simulink model "B2B_2x15kW_LCO_paralelo_y_serie"  (R2026b)
settings: Solver=ode5  StopTime=inf  EnableMultiTasking=on
StopFcn:
  | Modelo_Disable_B2B
undefined symbols (not defined in the file): ALPHA_DC, COS_RO, dataStateMachine, DiscIntNeverNeededParam, dq2abc, EN_G, getNormalizedOffset, I_MAX_G, INV_SIN_RO, KAW_CCG, KAW_DC, KI_CCG, KI_DC, KI_PLLG, KP_CCG, KP_DC, KP_PLLG, L12, LIMIT_SAG_DETECT, magnitude, MIN_VDC_READY, Ncount, NDELAY_SAG_DETECT, PORC_DC_STEADS, SAMPLES_SAG_DETECT, simDCcontCurrent1, simDCcontCurrent2, SN_G, Transformations_blocks, ts, Ts_al, TS_C, TS_PLL, UDC_min_al, UDC_Ref_al, VDC_REF, WN_G
libraries: simulink x15, TriPhaseDriveControl x13, powerlib_extras x2, model_hardware_PM15F80C_rev x2, TriphaseXenomaiTarget x1
(part 4 of 4)

== matlab function B2B_2x15kW_LCO_paralelo_y_serie/VSC2 Controller/State Machine/State Machine ==
  settings: fimath=|
      | fimath(...
      | 'RoundMode', 'floor',...
      | 'OverflowMode', 'wrap',...
      | 'ProductMode', 'KeepLSB', 'ProductWordLength', 32,...
      | 'SumMode', 'KeepLSB', 'SumWordLength', 32,...
      | 'CastBeforeSum', false)
  data: data input; outputs output; nowState output; nowCounters output; inputs input size=6; prevState input; prevCounters input
function [outputs, nowState, nowCounters] = fcn(data, inputs, prevState, prevCounters)

%%%%%%%%%%%%%%%%%%%%%%%%%%%%%%%%%%%%%%%%%%%%%%%%%%%%%%%%%%%%%%%%%%%%%%%%%%%
%List of states
%%%%%%%%%%%%%%%%%%%%%%%%%%%%%%%%%%%%%%%%%%%%%%%%%%%%%%%%%%%%%%%%%%%%%%%%%%%

%1: POWER_ON              : Power on, everything deactivated
%2: PRECHARGE             : Precharge of the DC-link capacitors
%3: STANDBY               : Waiting to start
%4: START                 : Start sequence 
%5: OPERATING             : Normal operation 

%Initial value
state = prevState;

%%%%%%%%%%%%%%%%%%%%%%%%%%%%%%%%%%%%%%%%%%%%%%%%%%%%%%%%%%%%%%%%%%%%%%%%%%%
%List of data
%%%%%%%%%%%%%%%%%%%%%%%%%%%%%%%%%%%%%%%%%%%%%%%%%%%%%%%%%%%%%%%%%%%%%%%%%%%

%1: Nprecharge
%2: Nconnect
%3: NinitCCG

%Set the data to variables
Nprecharge   = data(1);
Nconnect     = data(2);
NinitCCG     = data(3);

%%%%%%%%%%%%%%%%%%%%%%%%%%%%%%%%%%%%%%%%%%%%%%%%%%%%%%%%%%%%%%%%%%%%%%%%%%%
%List of Inputs
%%%%%%%%%%%%%%%%%%%%%%%%%%%%%%%%%%%%%%%%%%%%%%%%%%%%%%%%%%%%%%%%%%%%%%%%%%%

%1:  PRECHARGE         : 0 NO precharge required
%                      : 1 
%2:  CONNECT           : 0 NO connection required
%                      : 1
%3:  SEL_QVCONTROL     : 0 V controller
%                      : 1 Q controller
%4:  VDC_READY         : 0 VDV >= than stablished value
%                      : 1 
%5:  VDC_STEADS        : 0 Not reached DC steady-state
%                      : 1 
%6:  FLAG_SAG          : 0 No voltage sag detected
%                      : 1 

%Set the variables to its names
PRECHARGE     = inputs(1);
CONNECT       = inputs(2);
SEL_QVCONTROL = inputs(3);
VDC_READY     = inputs(4);
VDC_STEADS    = inputs(5);
FLAG_SAG      = inputs(6);

%%%%%%%%%%%%%%%%%%%%%%%%%%%%%%%%%%%%%%%%%%%%%%%%%%%%%%%%%%%%%%%%%%%%%%%%%%%
%List of outputs
%%%%%%%%%%%%%%%%%%%%%%%%%%%%%%%%%%%%%%%%%%%%%%%%%%%%%%%%%%%%%%%%%%%%%%%%%%%

%PWMOnGrid                     : 0 Do NOT PWM of grid converter
%                              : 1 
%CONNECT_GRID_CONTACT          : 0 NO connection to grid
%                              : 1
%CONNECT_PRELOAD_CONTACT       : 0 NO connection of precharge
%                              : 1 
%selReactiveVoltageController  : 0 Selection of V control
%                              : 1 Selection of Q control
%initPLLGrid                   : 0 Do NOT activate the PLL
%                              : 1 
%initReactiveVoltageController : 0 NO activate the external AC control (Q/VAC)
%                              : 1
%initCurrentControllerG        : 0 Do NOT initilialise the current controller
%                              : 1 
%initDCControllerGrid          : 0 Do NOT initialise the DC controller
%                              : 1                        

%Initilisation
PWMOnGrid               = 0;
CONNECT_GRID_CONTACT    = 0;
CONNECT_PRELOAD_CONTACT = 0;
selReactiveVoltageController  = SEL_QVCONTROL;
initPLLGrid             = 0;
initReactiveVoltageController = 0;
initCurrentControllerG  = 0;
initDCControllerGrid    = 0;

%%%%%%%%%%%%%%%%%%%%%%%%%%%%%%%%%%%%%%%%%%%%%%%%%%%%%%%%%%%%%%%%%%%%%%%%%%%
%List of counters
%%%%%%%%%%%%%%%%%%%%%%%%%%%%%%%%%%%%%%%%%%%%%%%%%%%%%%%%%%%%%%%%%%%%%%%%%%%

%Initilisation
CONT_PRECHARGE   = 0;
CONT_CONNECT     = 0;
CONT_INIT_CC     = 0;

%Adjustment of vector counters
CONT_PRECHARGE_ANT   = prevCounters(1);
CONT_CONNECT_ANT     = prevCounters(2);
CONT_INIT_CC_ANT     = prevCounters(3);

%%%%%%%%%%%%%%%%%%%%%%%%%%%%%%%%%%%%%%%%%%%%%%%%%%%%%%%%%%%%%%%%%%%%%%%%%%%
%STATE MACHINE: MAIN SWITCH
%%%%%%%%%%%%%%%%%%%%%%%%%%%%%%%%%%%%%%%%%%%%%%%%%%%%%%%%%%%%%%%%%%%%%%%%%%%

switch prevState

%%%%%%%%%%%%%%%%%%%%%%%%%%%%%%%%%%%%%%%%%%%%%%%%%%%%%%%%%%%%%%%%%%%%%%%%%%%
%STATE 1: POWER_ON
%%%%%%%%%%%%%%%%%%%%%%%%%%%%%%%%%%%%%%%%%%%%%%%%%%%%%%%%%%%%%%%%%%%%%%%%%%%

case 1

%Outputs for the state
PWMOnGrid               = 0;
CONNECT_GRID_CONTACT    = 0;
CONNECT_PRELOAD_CONTACT = 0;
selReactiveVoltageController  = SEL_QVCONTROL;
initPLLGrid             = 0;
initReactiveVoltageController = 0;
initDCControllerGrid    = 0;

%Counter initialisation
CONT_PRECHARGE   = 0;
CONT_CONNECT     = 0;
CONT_INIT_CC     = 0;

%Conditions to change state
if (PRECHARGE == 1) %Precharge
    state = 2;                            %Change to state 2 
end

%%%%%%%%%%%%%%%%%%%%%%%%%%%%%%%%%%%%%%%%%%%%%%%%%%%%%%%%%%%%%%%%%%%%%%%%%%%
%STATE 2: PRECHARGE
%%%%%%%%%%%%%%%%%%%%%%%%%%%%%%%%%%%%%%%%%%%%%%%%%%%%%%%%%%%%%%%%%%%%%%%%%%%

case 2

%Outputs for the state
PWMOnGrid               = 0;
CONNECT_GRID_CONTACT    = 0;
CONNECT_PRELOAD_CONTACT = 1;
selReactiveVoltageController = SEL_QVCONTROL;
initPLLGrid             = 1;
initReactiveVoltageController = 0;
initCurrentControllerG  = 0;
initDCControllerGrid    = 0;

%Counter initialisation
CONT_PRECHARGE   = 1;
CONT_CONNECT     = 0;
CONT_INIT_CC     = 0;

%Conditions to change state
if (PRECHARGE == 0) %If precharge is zero, go init
    state = 1;
end

if ((CONT_PRECHARGE_ANT >= Nprecharge) && (VDC_READY == 1)) % If time for precharge is reached
    state = 3;              %Go to standby
    CONT_PRECHARGE_ANT = 0; %Unload the counter
end

%%%%%%%%%%%%%%%%%%%%%%%%%%%%%%%%%%%%%%%%%%%%%%%%%%%%%%%%%%%%%%%%%%%%%%%%%%%
%STATE 3: STANDBY
%%%%%%%%%%%%%%%%%%%%%%%%%%%%%%%%%%%%%%%%%%%%%%%%%%%%%%%%%%%%%%%%%%%%%%%%%%%

case 3

%Outputs for the state
PWMOnGrid               = 0;
CONNECT_GRID_CONTACT    = 1;
CONNECT_PRELOAD_CONTACT = 0;
selReactiveVoltageController = SEL_QVCONTROL;
initPLLGrid             = 1;
initReactiveVoltageController = 0;
initCurrentControllerG  = 0;
initDCControllerGrid    = 0;

%Counter initialisation
CONT_PRECHARGE   = 0;
CONT_CONNECT     = 1;
CONT_INIT_CC     = 0;

%Conditions to change state
if ((CONT_CONNECT_ANT >= Nconnect) && (CONNECT == 1) && (VDC_STEADS == 1)) %If time to connect is reached
	state = 4; 
    CONT_CONNECT_ANT = 0; %Unload the counter
end

%%%%%%%%%%%%%%%%%%%%%%%%%%%%%%%%%%%%%%%%%%%%%%%%%%%%%%%%%%%%%%%%%%%%%%%%%%%
%STATE 4: START
%%%%%%%%%%%%%%%%%%%%%%%%%%%%%%%%%%%%%%%%%%%%%%%%%%%%%%%%%%%%%%%%%%%%%%%%%%%

case 4

%Outputs for the state
PWMOnGrid               = 1;
CONNECT_GRID_CONTACT    = 1;
CONNECT_PRELOAD_CONTACT = 0;
selReactiveVoltageController = SEL_QVCONTROL;
initPLLGrid             = 1;
initReactiveVoltageController = 0;
initCurrentControllerG  = 1;
initDCControllerGrid    = 1;

%Counter initialisation
CONT_PRECHARGE   = 0;
CONT_CONNECT     = 0;
CONT_INIT_CC     = 1;

%Conditions to change state
if (CONT_INIT_CC_ANT >= NinitCCG)  %If time to start is reached
    state = 5;                     %Go to regular operation
    CONT_INIT_CC_ANT = 0;          %Unload the counter
end

if (CONNECT == 0)  %If connect equals zero
    state = 1;     %Dischonnect
end

%%%%%%%%%%%%%%%%%%%%%%%%%%%%%%%%%%%%%%%%%%%%%%%%%%%%%%%%%%%%%%%%%%%%%%%%%%%
%STATE 5: OPERATING
%%%%%%%%%%%%%%%%%%%%%%%%%%%%%%%%%%%%%%%%%%%%%%%%%%%%%%%%%%%%%%%%%%%%%%%%%%%

case 5

%Outputs for the state
PWMOnGrid               = 1;
CONNECT_GRID_CONTACT    = 1;
CONNECT_PRELOAD_CONTACT = 0;
selReactiveVoltageController = SEL_QVCONTROL;
initPLLGrid             = 1;
initReactiveVoltageController = 1;
initCurrentControllerG  = 1;
initDCControllerGrid    = 1;

%Counter initialisation
CONT_PRECHARGE   = 0;
CONT_CONNECT     = 0;
CONT_INIT_CC     = 0;

%Conditions to change state
if (CONNECT == 0)  %If connect equals zero
    state = 1;     %Dischonnect
end

%%%%%%%%%%%%%%%%%%%%%%%%%%%%%%%%%%%%%%%%%%%%%%%%%%%%%%%%%%%%%%%%%%%%%%%%%%%
%STATE MACHINE: END STATE MACHINE
%%%%%%%%%%%%%%%%%%%%%%%%%%%%%%%%%%%%%%%%%%%%%%%%%%%%%%%%%%%%%%%%%%%%%%%%%%%

end 

%%%%%%%%%%%%%%%%%%%%%%%%%%%%%%%%%%%%%%%%%%%%%%%%%%%%%%%%%%%%%%%%%%%%%%%%%%%
%INCREASE AND RESET COUNTERS
%%%%%%%%%%%%%%%%%%%%%%%%%%%%%%%%%%%%%%%%%%%%%%%%%%%%%%%%%%%%%%%%%%%%%%%%%%%

%PRECHARGE counter
if (CONT_PRECHARGE == 1)
    CONT_PRECHARGE = CONT_PRECHARGE_ANT + CONT_PRECHARGE;
else
    CONT_PRECHARGE = 0;
end

%CONNECT counter
if (CONT_CONNECT == 1)
    CONT_CONNECT = CONT_CONNECT_ANT + CONT_CONNECT;
else
    CONT_CONNECT = 0;
end

%INIT_CC counter
if (CONT_INIT_CC == 1)
    CONT_INIT_CC = CONT_INIT_CC_ANT + CONT_INIT_CC;
else
    CONT_INIT_CC = 0;
end

%%%%%%%%%%%%%%%%%%%%%%%%%%%%%%%%%%%%%%%%%%%%%%%%%%%%%%%%%%%%%%%%%%%%%%%%%%%
%OUTPUT GENERATOR
%%%%%%%%%%%%%%%%%%%%%%%%%%%%%%%%%%%%%%%%%%%%%%%%%%%%%%%%%%%%%%%%%%%%%%%%%%%

%Vector of outputs
outputs = [PWMOnGrid CONNECT_GRID_CONTACT CONNECT_PRELOAD_CONTACT selReactiveVoltageController initPLLGrid initReactiveVoltageController initCurrentControllerG initDCControllerGrid]';

%Vector of outputs
nowState = state;

%Vector with new counters
nowCounters = [CONT_PRECHARGE CONT_CONNECT CONT_INIT_CC]';
